simulink model "InverterModel_HighFidelity"  (R2019a)
settings: Solver=VariableStepAuto  StartTime=0.0  StopTime=10.0  RelTol=1e-3
values from neighbouring files (symbols this model uses):
  J = 0.10    (= 0.1)    [DriveTrainInitialise.m]
  Tmax = 50    [DriveTrainInitialise.m]
  Ts = 2e-6    (= 2e-06)    [DriveTrainInitialise.m]
  Tsc = 1/fc    (= 5e-05)    [DriveTrainInitialise.m]
libraries: ee_lib x8, nesl_utility x8, fl_lib x2, eePmsmFieldOrientedControl x1
settings Model: Creator=plewi  LastModifiedBy=plewi

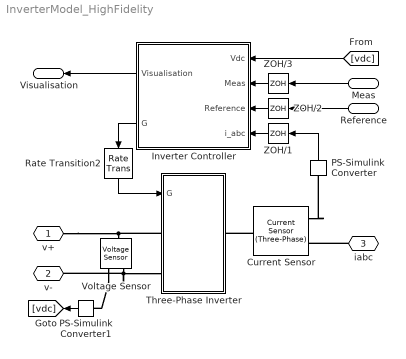
== system InverterModel_HighFidelity ==
  Reference : Inport
  Meas : Inport  Port=2
  Current Sensor : ee_lib/Sensors & Transducers/Current Sensor (Three-Phase)
      settings: SourceProductName=Simscape Electrical
  Inverter Controller : Subsystem
  PS-Simulink Converter : nesl_utility/PS-Simulink Converter  PhysicalDomain=network_engine_domain  SubClassName=ps_output  LeftPortType=input  RightPortType=output  PseudoPeriodic=off  Frequencies=[]  Unit=1  AffineConversion=off
  PS-Simulink Converter1 : nesl_utility/PS-Simulink Converter  PhysicalDomain=network_engine_domain  SubClassName=ps_output  LeftPortType=input  RightPortType=output  PseudoPeriodic=off  Frequencies=[]  Unit=1  AffineConversion=off
  Rate Transition2 : RateTransition  OutPortSampleTime=Ts
  Three-Phase Inverter : Subsystem
  Voltage Sensor : fl_lib/Electrical/Electrical Sensors/Voltage Sensor
  ZOH/1 : ZeroOrderHold  SampleTime=Tsc
  ZOH/2 : ZeroOrderHold  SampleTime=Tsc
  ZOH/3 : ZeroOrderHold  SampleTime=Tsc
  v+ : PMIOPort  Side=Left
  v- : PMIOPort  Port=2  Side=Left
  iabc : PMIOPort  Port=3  Side=Left
  Visualisation : Outport  Port=3
  wires:
  PS-Simulink Converter/1 -> ZOH/1/1
  Rate Transition2/1 -> Three-Phase Inverter/1(G)
  Meas/1 -> ZOH/3/1
  Inverter Controller/2(G) -> Rate Transition2/1
  [vdc] -> Inverter Controller/1(Vdc)
  ZOH/2/1 -> Inverter Controller/3(Reference)
  ZOH/3/1 -> Inverter Controller/2(Meas)
  ZOH/1/1 -> Inverter Controller/4(i_abc)
  Reference/1 -> ZOH/2/1
  PS-Simulink Converter1/1 -> [vdc]
  Inverter Controller/1(Visualisation) -> Visualisation/1
  connections:
  Current Sensor/LConn1 -- Three-Phase Inverter/RConn1
  Current Sensor/RConn1 -- PS-Simulink Converter/LConn1
  Three-Phase Inverter/LConn1 -- v+/RConn1 -- Voltage Sensor/LConn1
  Voltage Sensor/RConn2 -- v-/RConn1 -- Three-Phase Inverter/LConn2
  Voltage Sensor/RConn1 -- PS-Simulink Converter1/LConn1
  iabc/RConn1 -- Current Sensor/RConn2

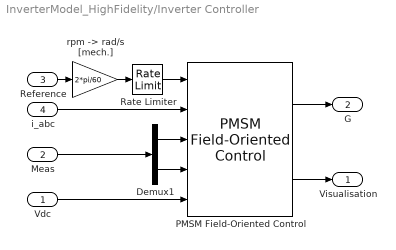
== system InverterModel_HighFidelity/Inverter Controller ==
  Vdc : Inport
  Meas : Inport  Port=2
  Reference : Inport  Port=3
  i_abc : Inport  Port=4
  Demux1 : Demux  Outputs=2
  PMSM Field-Oriented Control : eePmsmFieldOrientedControl/PMSM Field-Oriented Control  CtrlMode=Velocity control  Vnom=Vnom  Pmax=Pmax  Tmax=Tmax*1.5  p=PolePairs  Vdc_on=10  Ts=Ts  Tsc=Tsc  CtrlType=PI control  Kp_w=50  Ki_w=500  Kv_w=1  Kaw_w=1000  RefType=Zero d-axis control  rpmVec=[0, 3000]  TqVec=[-100, 0, 100]  VdcVec=[300, 350]  idMatrix=zeros(2,3,2)  iqMatrix=zeros(2,3,2)  psim=PM  Ld=0.00024  Lq=0.00029  Rs=0.01  AxisAlignment=Q-axis  Kp_id=0.6  Ki_id=6  Kaw_id=100  Kp_iq=0.2  Ki_iq=8  Kaw_iq=100  AxisPrio=Q-axis  ActZC=off  ActFF=on  ParamTypeFF=Constant parameters  LdFF=Ld  LqFF=Lq  psimFF=PM  idVect=[-200, 0, 200]  iqVect=[-200, 0, 200]  LdMatrix=0.0002 * ones(3, 3)  LqMatrix=0.0002 * ones(3, 3)  psimMatrix=0.04 * ones(3, 3)  CPWMMode=SVM: space vector modulation  fsw=fsw
      settings: SourceProductName=Simscape Electrical  SourceProductBaseCode=PS
  Rate Limiter : RateLimiter  RisingSlewLimit=Tmax/J  FallingSlewLimit=-Tmax/J  SampleTimeMode=inherited
  "rpm -> rad/s [mech.]" : Gain  Gain=2*pi/60
  Visualisation : Outport
  G : Outport  Port=2
  wires:
  PMSM Field-Oriented Control/1 -> G/1
  Vdc/1 -> PMSM Field-Oriented Control/5
  PMSM Field-Oriented Control/2 -> Visualisation/1
  i_abc/1 -> PMSM Field-Oriented Control/2
  Meas/1 -> Demux1/1
  Demux1/1 -> PMSM Field-Oriented Control/3
  Demux1/2 -> PMSM Field-Oriented Control/4
  Reference/1 -> "rpm -> rad/s [mech.]"/1
  Rate Limiter/1 -> PMSM Field-Oriented Control/1
  "rpm -> rad/s [mech.]"/1 -> Rate Limiter/1

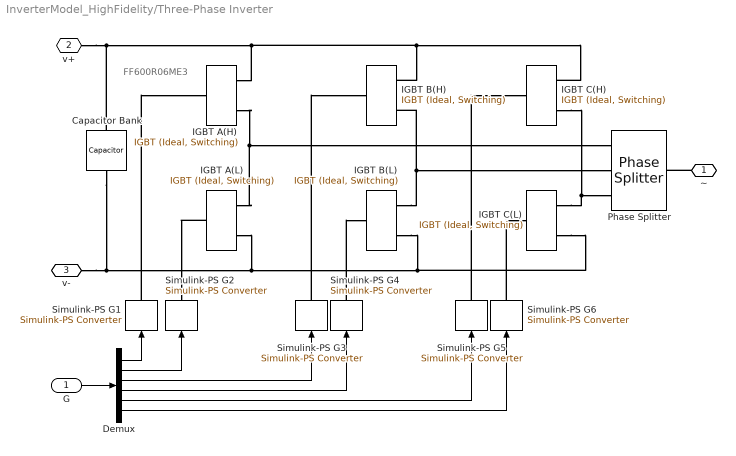
== system InverterModel_HighFidelity/Three-Phase Inverter ==
  note: FF600R06ME3
  G : Inport
  Capacitor Bank : fl_lib/Electrical/Electrical Elements/Capacitor  c=1e-1 F  r=0 Ohm  g=0 1/Ohm  i_specify=off  i_priority=None  i=0 A  i_nominal_specify=off  i_nominal_unit=A  i_nominal_value=1  v_specify=off  v_priority=None  v=0 V  v_nominal_specify=off  v_nominal_unit=V  v_nominal_value=1  vc_specify=off  vc_priority=High  vc=0 V  vc_nominal_specify=off  vc_nominal_unit=V  vc_nominal_value=1
  Demux : Demux  Outputs=6
  IGBT A(H) : ee_lib/Semiconductors & Converters/IGBT (Ideal, Switching)  Description=Bamocar D3 IGBT Model Number: FF600R06ME3  Vf=Vf V  Ron=Ron Ohm  Goff=Goff S  Vth=Vth V  diode_param=2  diode_Vf=Vf_diode V  diode_Ron=Ron_diode Ohm  diode_Goff=Goff_diode S  diode_C=5e-8 F  diode_iRM=-235 A  diode_iF=300 A  diode_idot=-50 A/us  diode_trr_param=1  diode_trr_factor=3  diode_trr=15 us  diode_Qrr=1.5e+3 s*uA  thermal_loss_option=2  Voff=300 V  Tau=1e-4 s  Tj=[298.15, 398.15] K  Iout_scalar=600 A  Eon_scalar=22.86e-3 J  Eoff_scalar=17.14e-3 J  Von_scalar=2.7 V  Iout_data=[0, 10, 50, 100, 200, 400, 600] A  Eon_data=[0, .29, 1.43, 2.86, 5.71, 13.14, 22.86; 0, .57, 2.63, 5.14, 10.29, 20.57, 30.29] * 1e-3 J  Eoff_data=[0, .21, 1.07, 2.14, 4.29, 9.86, 17.14; 0, .43, 1.97, 3.86, 7.71, 15.43, 22.71] * 1e-3 J  Von_data=[0, 1.1, 1.3, 1.45, 1.75, 2.25, 2.7; 0, 1, 1.15, 1.35, 1.7, 2.35, 3] V
      settings: SourceProductName=Simscape Electrical
  IGBT A(L) : ee_lib/Semiconductors & Converters/IGBT (Ideal, Switching)  Description=Bamocar D3 IGBT Model Number: FF600R06ME3  Vf=Vf V  Ron=Ron Ohm  Goff=Goff S  Vth=Vth V  diode_param=2  diode_Vf=Vf_diode V  diode_Ron=Ron_diode Ohm  diode_Goff=Goff_diode S  diode_C=5e-8 F  diode_iRM=-235 A  diode_iF=300 A  diode_idot=-50 A/us  diode_trr_param=1  diode_trr_factor=3  diode_trr=15 us  diode_Qrr=1.5e+3 s*uA  thermal_loss_option=2  Voff=300 V  Tau=1e-4 s  Tj=[298.15, 398.15] K  Iout_scalar=600 A  Eon_scalar=22.86e-3 J  Eoff_scalar=17.14e-3 J  Von_scalar=2.7 V  Iout_data=[0, 10, 50, 100, 200, 400, 600] A  Eon_data=[0, .29, 1.43, 2.86, 5.71, 13.14, 22.86; 0, .57, 2.63, 5.14, 10.29, 20.57, 30.29] * 1e-3 J  Eoff_data=[0, .21, 1.07, 2.14, 4.29, 9.86, 17.14; 0, .43, 1.97, 3.86, 7.71, 15.43, 22.71] * 1e-3 J  Von_data=[0, 1.1, 1.3, 1.45, 1.75, 2.25, 2.7; 0, 1, 1.15, 1.35, 1.7, 2.35, 3] V
      settings: SourceProductName=Simscape Electrical
  IGBT B(H) : ee_lib/Semiconductors & Converters/IGBT (Ideal, Switching)  Description=Bamocar D3 IGBT Model Number: FF600R06ME3  Vf=Vf V  Ron=Ron Ohm  Goff=Goff S  Vth=Vth V  diode_param=2  diode_Vf=Vf_diode V  diode_Ron=Ron_diode Ohm  diode_Goff=Goff_diode S  diode_C=5e-8 F  diode_iRM=-235 A  diode_iF=300 A  diode_idot=-50 A/us  diode_trr_param=1  diode_trr_factor=3  diode_trr=15 us  diode_Qrr=1.5e+3 s*uA  thermal_loss_option=2  Voff=300 V  Tau=1e-4 s  Tj=[298.15, 398.15] K  Iout_scalar=600 A  Eon_scalar=22.86e-3 J  Eoff_scalar=17.14e-3 J  Von_scalar=2.7 V  Iout_data=[0, 10, 50, 100, 200, 400, 600] A  Eon_data=[0, .29, 1.43, 2.86, 5.71, 13.14, 22.86; 0, .57, 2.63, 5.14, 10.29, 20.57, 30.29] * 1e-3 J  Eoff_data=[0, .21, 1.07, 2.14, 4.29, 9.86, 17.14; 0, .43, 1.97, 3.86, 7.71, 15.43, 22.71] * 1e-3 J  Von_data=[0, 1.1, 1.3, 1.45, 1.75, 2.25, 2.7; 0, 1, 1.15, 1.35, 1.7, 2.35, 3] V
      settings: SourceProductName=Simscape Electrical
  IGBT B(L) : ee_lib/Semiconductors & Converters/IGBT (Ideal, Switching)  Description=Bamocar D3 IGBT Model Number: FF600R06ME3  Vf=Vf V  Ron=Ron Ohm  Goff=Goff S  Vth=Vth V  diode_param=2  diode_Vf=Vf_diode V  diode_Ron=Ron_diode Ohm  diode_Goff=Goff_diode S  diode_C=5e-8 F  diode_iRM=-235 A  diode_iF=300 A  diode_idot=-50 A/us  diode_trr_param=1  diode_trr_factor=3  diode_trr=15 us  diode_Qrr=1.5e+3 s*uA  thermal_loss_option=2  Voff=300 V  Tau=1e-4 s  Tj=[298.15, 398.15] K  Iout_scalar=600 A  Eon_scalar=22.86e-3 J  Eoff_scalar=17.14e-3 J  Von_scalar=2.7 V  Iout_data=[0, 10, 50, 100, 200, 400, 600] A  Eon_data=[0, .29, 1.43, 2.86, 5.71, 13.14, 22.86; 0, .57, 2.63, 5.14, 10.29, 20.57, 30.29] * 1e-3 J  Eoff_data=[0, .21, 1.07, 2.14, 4.29, 9.86, 17.14; 0, .43, 1.97, 3.86, 7.71, 15.43, 22.71] * 1e-3 J  Von_data=[0, 1.1, 1.3, 1.45, 1.75, 2.25, 2.7; 0, 1, 1.15, 1.35, 1.7, 2.35, 3] V
      settings: SourceProductName=Simscape Electrical
  IGBT C(H) : ee_lib/Semiconductors & Converters/IGBT (Ideal, Switching)  Description=Bamocar D3 IGBT Model Number: FF600R06ME3  Vf=Vf V  Ron=Ron Ohm  Goff=Goff S  Vth=Vth V  diode_param=2  diode_Vf=Vf_diode V  diode_Ron=Ron_diode Ohm  diode_Goff=Goff_diode S  diode_C=5e-8 F  diode_iRM=-235 A  diode_iF=300 A  diode_idot=-50 A/us  diode_trr_param=1  diode_trr_factor=3  diode_trr=15 us  diode_Qrr=1.5e+3 s*uA  thermal_loss_option=2  Voff=300 V  Tau=1e-4 s  Tj=[298.15, 398.15] K  Iout_scalar=600 A  Eon_scalar=22.86e-3 J  Eoff_scalar=17.14e-3 J  Von_scalar=2.7 V  Iout_data=[0, 10, 50, 100, 200, 400, 600] A  Eon_data=[0, .29, 1.43, 2.86, 5.71, 13.14, 22.86; 0, .57, 2.63, 5.14, 10.29, 20.57, 30.29] * 1e-3 J  Eoff_data=[0, .21, 1.07, 2.14, 4.29, 9.86, 17.14; 0, .43, 1.97, 3.86, 7.71, 15.43, 22.71] * 1e-3 J  Von_data=[0, 1.1, 1.3, 1.45, 1.75, 2.25, 2.7; 0, 1, 1.15, 1.35, 1.7, 2.35, 3] V
      settings: SourceProductName=Simscape Electrical
  IGBT C(L) : ee_lib/Semiconductors & Converters/IGBT (Ideal, Switching)  Description=Bamocar D3 IGBT Model Number: FF600R06ME3  Vf=Vf V  Ron=Ron Ohm  Goff=Goff S  Vth=Vth V  diode_param=2  diode_Vf=Vf_diode V  diode_Ron=Ron_diode Ohm  diode_Goff=Goff_diode S  diode_C=5e-8 F  diode_iRM=-235 A  diode_iF=300 A  diode_idot=-50 A/us  diode_trr_param=1  diode_trr_factor=3  diode_trr=15 us  diode_Qrr=1.5e+3 s*uA  thermal_loss_option=2  Voff=300 V  Tau=1e-4 s  Tj=[298.15, 398.15] K  Iout_scalar=600 A  Eon_scalar=22.86e-3 J  Eoff_scalar=17.14e-3 J  Von_scalar=2.7 V  Iout_data=[0, 10, 50, 100, 200, 400, 600] A  Eon_data=[0, .29, 1.43, 2.86, 5.71, 13.14, 22.86; 0, .57, 2.63, 5.14, 10.29, 20.57, 30.29] * 1e-3 J  Eoff_data=[0, .21, 1.07, 2.14, 4.29, 9.86, 17.14; 0, .43, 1.97, 3.86, 7.71, 15.43, 22.71] * 1e-3 J  Von_data=[0, 1.1, 1.3, 1.45, 1.75, 2.25, 2.7; 0, 1, 1.15, 1.35, 1.7, 2.35, 3] V
      settings: SourceProductName=Simscape Electrical
  Phase Splitter : ee_lib/Connectors & References/Phase Splitter
      settings: SourceProductName=Simscape Electrical  SourceProductBaseCode=PS
  Simulink-PS G{1..6} (6 alike) : nesl_utility/Simulink-PS Converter  PhysicalDomain=network_engine_domain  SubClassName=ps_input  LeftPortType=input  RightPortType=output  PseudoPeriodic=off  Frequencies=[]  NoiseDistribution=none  NoiseParameters=[]  Unit=1  AffineConversion=off  FilteringAndDerivatives=zero  SimscapeFilterOrder=1  InputFilterTimeConstant=1e-6  UdotUserProvided=0
  ~ : PMIOPort  Tag=PMCPort  Side=Right
  v+ : PMIOPort  Tag=PMCPort  Port=2  Side=Left
  v- : PMIOPort  Tag=PMCPort  Port=3  Side=Left
  wires:
  Demux/6 -> Simulink-PS G6/1
  Demux/5 -> Simulink-PS G5/1
  Demux/4 -> Simulink-PS G4/1
  Demux/3 -> Simulink-PS G3/1
  Demux/2 -> Simulink-PS G2/1
  G/1 -> Demux/1
  Demux/1 -> Simulink-PS G1/1
  connections:
  Simulink-PS G6/RConn1 -- IGBT C(L)/LConn1
  Simulink-PS G5/RConn1 -- IGBT C(H)/LConn1
  Simulink-PS G4/RConn1 -- IGBT B(L)/LConn1
  Simulink-PS G3/RConn1 -- IGBT B(H)/LConn1
  IGBT A(L)/LConn1 -- Simulink-PS G2/RConn1
  IGBT B(L)/RConn2 -- Capacitor Bank/RConn1 -- v-/RConn1 -- IGBT A(L)/RConn2 -- IGBT C(L)/RConn2
  IGBT A(H)/RConn2 -- Phase Splitter/RConn1 -- IGBT A(L)/RConn1
  IGBT B(L)/RConn1 -- Phase Splitter/RConn2 -- IGBT B(H)/RConn2
  IGBT C(L)/RConn1 -- Phase Splitter/RConn3 -- IGBT C(H)/RConn2
  IGBT B(H)/RConn1 -- Capacitor Bank/LConn1 -- v+/RConn1 -- IGBT A(H)/RConn1 -- IGBT C(H)/RConn1
  ~/RConn1 -- Phase Splitter/LConn1
  Simulink-PS G1/RConn1 -- IGBT A(H)/LConn1
